simulink model "Journal2022"  (R2018a)
settings: Solver=VariableStepAuto  StartTime=0.0  StopTime=20  FixedStep=1e-6  MinStep=1e-3  RelTol=1e-3  EnableMultiTasking=on
PreLoadFcn:
  | if count(py.sys.path,'') == 0
  | insert(py.sys.path,int32(0),'');
  | end
InitFcn:
  | clear all
  | close all
  | Variables_Journal2022
StopFcn:
  | %Figures_Test_Pytorch_simulink
values from neighbouring files (symbols this model uses):
  den_Tdel = [0 0.2]    [TestKalm.mat]    (also in Variables_Journal2022.m)
  Fz_routa = 7840    [TestKalm.mat]    (also in Variables_Journal2022.m)
  G1 = -4.99    [Variables_Journal2022.m]
  G2 = -18.43    [Variables_Journal2022.m]
  G3 = -65.62    [Variables_Journal2022.m]
  lambda_dummy = [0 0.000200040008002 0.000400080016003 0.000600120024005 0.000800160032006 0.00100020004001 0.00120024004801 0.00140028005601 0.00160032006401 0.00180036007201 0.00200040008002 0.00220044008802 ... (5000 elements, 1x5000)]    [TestKalm.mat]    (also in Variables_Journal2022.m = linspace(0, 1, num_samples_lambda))
  Massa_drone_eq = 800    [TestKalm.mat]    (also in Variables_Journal2022.m)
  ML_sample_time = 0.005    [TestKalm.mat]    (also in Variables_Journal2022.m)
  Momento_inerzia = 0.45    [TestKalm.mat]    (also in Variables_Journal2022.m)
  omega0 = 266.666666667    [TestKalm.mat]    (also in Variables_Journal2022.m)
  PI_ki = 20    [TestKalm.mat]    (also in Variables_Journal2022.m)
  PI_kp = 0.5    [TestKalm.mat]    (also in Variables_Journal2022.m)
  Raggio_pneumatico = 0.3    [TestKalm.mat]    (also in Variables_Journal2022.m)
  Sample_time = 0.005    [TestKalm.mat]    (also in Variables_Journal2022.m)
  v0 = 80    [TestKalm.mat]    (also in Variables_Journal2022.m)
  v_min_stop = 15    [Variables_Journal2022.m]
  v_state_space_A = [-200  -10000; 1  0]    [TestKalm.mat]    (also in Variables_Journal2022.m = Av)
  v_state_space_B = [1 0]    [TestKalm.mat]    (also in Variables_Journal2022.m = Bv)
  v_state_space_C = [10000  0; 1  0; 0  1]    [TestKalm.mat]    (also in Variables_Journal2022.m = [Cv; eye(2)])
  v_state_space_D = [0 0 0]    [TestKalm.mat]    (also in Variables_Journal2022.m = [Dv; 0;0])
  v_state_space_init = [0 0.008]    [TestKalm.mat]    (also in Variables_Journal2022.m = [inv(Av)*-Bv*v0])
  w_state_Space_A = [-200  -10000; 1  0]    [TestKalm.mat]    (also in Variables_Journal2022.m = Aw)
  w_state_Space_B = [1 0]    [TestKalm.mat]    (also in Variables_Journal2022.m = Bw)
  w_state_Space_C = [10000  0; 1  0; 0  1]    [TestKalm.mat]    (also in Variables_Journal2022.m = [Cw; eye(2)])
  w_state_Space_D = [0 0 0]    [TestKalm.mat]    (also in Variables_Journal2022.m = [Dw; 0;0])
  w_state_space_init = [0 0.0266666666667]    [TestKalm.mat]    (also in Variables_Journal2022.m = [inv(Aw)*-Bw*omega0])
undefined symbols (not defined in the file or in its folder): sigbuilder_block
libraries: simulink x5, ctrlSharedLib x1
settings Model: Creator=Francesco  LastModifiedBy=Francesco Crocetti
settings DataIOCC: LimitDataPoints=on  SaveFormat=Array
settings OptimizationCC: LifeSpan=inf
settings DebuggingCC: SolverPrmCheckMsg=warning  SFUnexpectedBacktrackingDiag=warning  SFNoUnconditionalDefaultTransitionDiag=warning  SFExecutionAtInitializationDiag=none
settings HardwareCC: ProdBitPerPointer=32  ProdBitPerSizeT=32  ProdBitPerPtrDiffT=32  ProdLargestAtomicFloat=None  ProdIntDivRoundTo=Undefined  ProdEndianess=Unspecified  ProdWordSize=32  ProdHWDeviceType=32-bit Generic
settings ModelReferenceCC: PropagateSignalLabelsOutOfModel=off
settings CodeAppCC: StateflowObjectComments=on
settings GRTTargetCC: TargetLangStandard=C89/C90 (ANSI)  GeneratePreprocessorConditionals=Disable all
settings ConfigComp: CovMetricSettings=dw  CovHtmlReporting=on  CovSaveCumulativeToWorkspaceVar=on  CovSaveSingleToWorkspaceVar=on  CovExternalEMLEnable=off  CovSFcnEnable=off

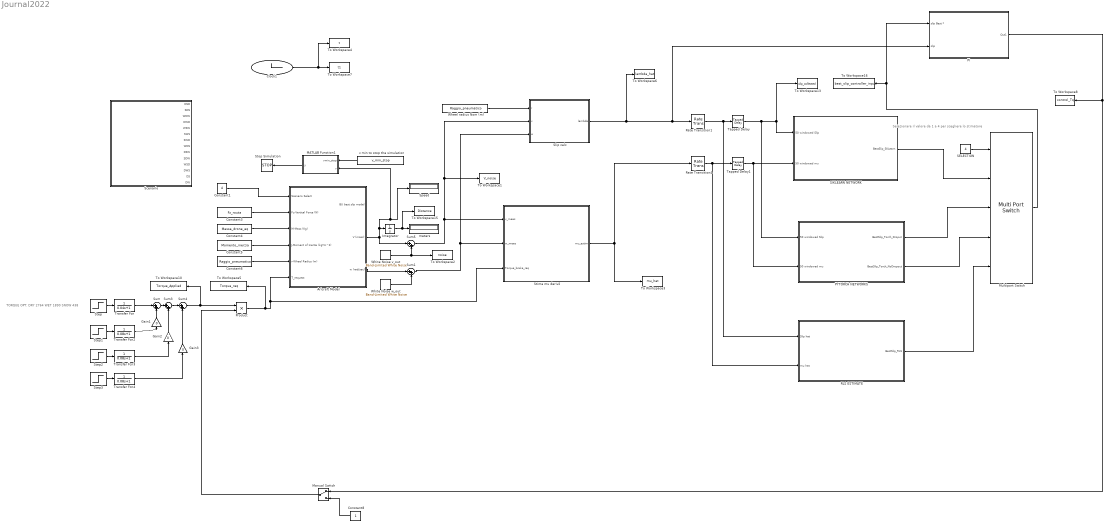
== system Journal2022 ==
  note: TORQUE OPT: DRY 2764 WET 1890 SNOW 438
  note: Selezionare il valore da 1 a 4 per scegliere lo stimatore
  Aricraft Model : Subsystem
  Clock1 : Clock
  Constant1 : Constant  Value=4
  Constant3 : Constant  Value=Fz_routa
  Constant4 : Constant  Value=Massa_drone_eq
  Constant5 : Constant  Value=Momento_inerzia
  Constant6 : Constant  Value=Raggio_pneumatico
  Constant8 : Constant
  Gain1 : Gain  Gain=0
  Gain2 : Gain  Gain=0
  Gain3 : Gain  Gain=0
  Integrator : Integrator
  MATLAB Function1 : MATLAB Function  TreatAsAtomicUnit=on
  Manual Switch : ManualSwitch
  Multiport Switch : MultiPortSwitch  DataPortOrder=Specify indices  Inputs=4  DataPortIndices={1,2,3,4}  DiagnosticForDefault=None  OutDataTypeStr=double  RndMeth=Round
  "PI " : Subsystem
  PYTORCH NETWORKS : Subsystem
  Product : Product
  RLS ESTIMATE : Subsystem
  Rate Transition1 : RateTransition  OutPortSampleTime=ML_sample_time
  Rate Transition4 : RateTransition  OutPortSampleTime=ML_sample_time
  SELECTION : Constant  Value=4
  SIKLEARN NETWORK : Subsystem
  "Scenario " : Subsystem  Tag=STV Subsys  LoadFcn=sigbuilder_block('load');  StartFcn=sigbuilder_block('start');  StopFcn=sigbuilder_block('stop');  ClipboardFcn=sigbuilder_block('clipboard');  mask(Sigbuilder block){tuvar=[0:10]}
      mask help: Simulink:masks:SigbuilderBlock_MD
      mask init:
      | if ~strcmp(get_param(bdroot(gcbh),'SimulationStatus'),'stopped') tuvar = sigbuilder_block('maskInit'); end
      settings: CopyFcn=sigbuilder_block('copy');  DeleteFcn=sigbuilder_block('delete');  ModelCloseFcn=sigbuilder_block('modelClose');  PreSaveFcn=sigbuilder_block('preSave');  PauseFcn=sigbuilder_block('pause');  ContinueFcn=sigbuilder_block('continue');  NameChangeFcn=sigbuilder_block('namechange');  OpenFcn=sigbuilder_block('open',[48.75 0 1391.25 690 ]);  CloseFcn=sigbuilder_block('close');
      mask Display: plot(0, 0, 100, 100,[2, 2, 32, 32, 2], [68, 8, 8, 68, 68],[32, 2], [38, 38], [32, 19, 2],[53, 60, 44], [32, 17, 17, 2],[16, 16, 31, 31]);txt = getActiveGroup(gcbh);text(2, 100, txt,'verticalAlignment', 'top');
  Slip calc : MATLAB Function  TreatAsAtomicUnit=on
  Speed : Display
  Step : Step  Time=0  After=3764  SampleTime=0
  Step1 : Step  Time=2  After=-500  SampleTime=0
  Step2 : Step  Time=4  After=-500  SampleTime=0
  Step3 : Step  Time=6  After=-500  SampleTime=0
  Stima mu deriv2 : Subsystem
  Stop Simulation : Stop
  Sum{,1,3..5} (5 alike) : Sum  Inputs=|++
  Tapped Delay : simulink/Discrete/Tapped Delay  vinit=0.2  samptime=-1  NumDelays=50  DelayOrder=Newest  includeCurrent=off
  Tapped Delay1 : simulink/Discrete/Tapped Delay  vinit=1  samptime=-1  NumDelays=50  DelayOrder=Newest  includeCurrent=off
  To Workspace1 : ToWorkspace  VariableName=V_noise  SampleTime=-1
  To Workspace10 : ToWorkspace  VariableName=Torque_Applied  SampleTime=-1
  To Workspace13 : ToWorkspace  VariableName=slip_collected  SampleTime=-1
  To Workspace15 : ToWorkspace  VariableName=Distance  SampleTime=-1
  To Workspace16 : ToWorkspace  VariableName=best_slip_controller_input  SampleTime=-1
  To Workspace2 : ToWorkspace  VariableName=noise  SampleTime=-1
  To Workspace3 : ToWorkspace  VariableName=mu_hat  SampleTime=-1
  To Workspace4 : ToWorkspace  VariableName=t  SampleTime=-1
  To Workspace5 : ToWorkspace  VariableName=Torque_req  SampleTime=-1
  To Workspace6 : ToWorkspace  VariableName=lambda_hat  SampleTime=-1
  To Workspace7 : ToWorkspace  VariableName=t1  SampleTime=Sample_time
  To Workspace8 : ToWorkspace  VariableName=control_Tq  SampleTime=-1
  Transfer Fcn : TransferFcn  Denominator=[0.04 1]
  Transfer Fcn2 : TransferFcn  Denominator=[0.08 1]
  Transfer Fcn3 : TransferFcn  Denominator=[0.08 1]
  Transfer Fcn4 : TransferFcn  Denominator=[0.08 1]
  Wheel radius Nom (m) : Constant  Value=Raggio_pneumatico
  White Noise v_out : simulink/Sources/Band-Limited White Noise  Cov=Pow_WN_vout_model  Ts=Sample_time  seed=[75893]
  White Noise w_out : simulink/Sources/Band-Limited White Noise  Cov=Pow_WN_wout_model  Ts=Sample_time  seed=[17523]
  meters : Display
  v min to stop the simulation : Constant  Value=v_min_stop
  wires:
  Integrator/1 -> To Workspace15/1, meters/1
  Constant6/1 -> Aricraft Model/5(r-Wheel Radius (m))
  Wheel radius Nom (m)/1 -> Slip calc/1(r)
  Constant4/1 -> Aricraft Model/3(" M-Mass (Kg)")
  Constant5/1 -> Aricraft Model/4(J-Moment of Inertia (‎kg*m^2))
  Sum5/1 -> Stima mu deriv2/1(v_meas), To Workspace1/1, Slip calc/2(v)
  Rate Transition4/1 -> RLS ESTIMATE/2(mu hat), Tapped Delay1/1
  Aricraft Model/3(w (rad/sec)) -> Sum1/1
  Sum1/1 -> Stima mu deriv2/2(w_meas), Slip calc/3(w)
  Clock1/1 -> To Workspace7/1, To Workspace4/1
  Transfer Fcn/1 -> Sum/1
  Step/1 -> Transfer Fcn/1
  Sum3/1 -> Sum4/1
  Transfer Fcn2/1 -> Gain1/1
  Step1/1 -> Transfer Fcn2/1
  Step2/1 -> Transfer Fcn3/1
  Transfer Fcn4/1 -> Gain3/1
  Transfer Fcn3/1 -> Gain2/1
  Sum/1 -> Sum3/1
  Step3/1 -> Transfer Fcn4/1
  Stima mu deriv2/1("mu_estim ") -> To Workspace3/1, Rate Transition4/1
  Slip calc/1(lambda) -> To Workspace6/1, "PI "/2("slip "), Rate Transition1/1
  Sum4/1 -> To Workspace10/1, Product/1
  Gain1/1 -> Sum/2
  Gain2/1 -> Sum3/2
  Gain3/1 -> Sum4/2
  Constant3/1 -> Aricraft Model/2(Fz-Vertical Force (N))
  Tapped Delay/1 -> PYTORCH NETWORKS/1(50 windowed Slip), SIKLEARN NETWORK/1(50 windowed Slip), To Workspace13/1
  White Noise v_out/1 -> Sum5/2, To Workspace2/1
  White Noise w_out/1 -> Sum1/2
  Tapped Delay1/1 -> SIKLEARN NETWORK/2(50 windowed mu), PYTORCH NETWORKS/2(50 windowed mu)
  Product/1 -> To Workspace5/1, Stima mu deriv2/3(Torque_brake_req), Aricraft Model/6(T_request)
  Rate Transition1/1 -> RLS ESTIMATE/1(" Slip hat"), Tapped Delay/1
  Constant8/1 -> Manual Switch/2
  Manual Switch/1 -> Product/2
  "PI "/1(Out1) -> Manual Switch/1, To Workspace8/1
  Multiport Switch/1 -> To Workspace16/1, "PI "/1("slip Best * ")
  PYTORCH NETWORKS/1(BestSlip_Torch_Droput) -> Multiport Switch/3
  PYTORCH NETWORKS/2(BestSlip_Torch_NoDropout) -> Multiport Switch/4
  MATLAB Function1/1(y) -> Stop Simulation/1
  Aricraft Model/2(V (msec)) -> Sum5/1, MATLAB Function1/2(v), Speed/1, Integrator/1
  v min to stop the simulation/1 -> MATLAB Function1/1(vmin_stop)
  RLS ESTIMATE/1("BestSlip_RLS ") -> Multiport Switch/5
  SELECTION/1 -> Multiport Switch/1
  SIKLEARN NETWORK/1(BestSlip_SKLearn) -> Multiport Switch/2
  Constant1/1 -> Aricraft Model/1("Scenario Select ")

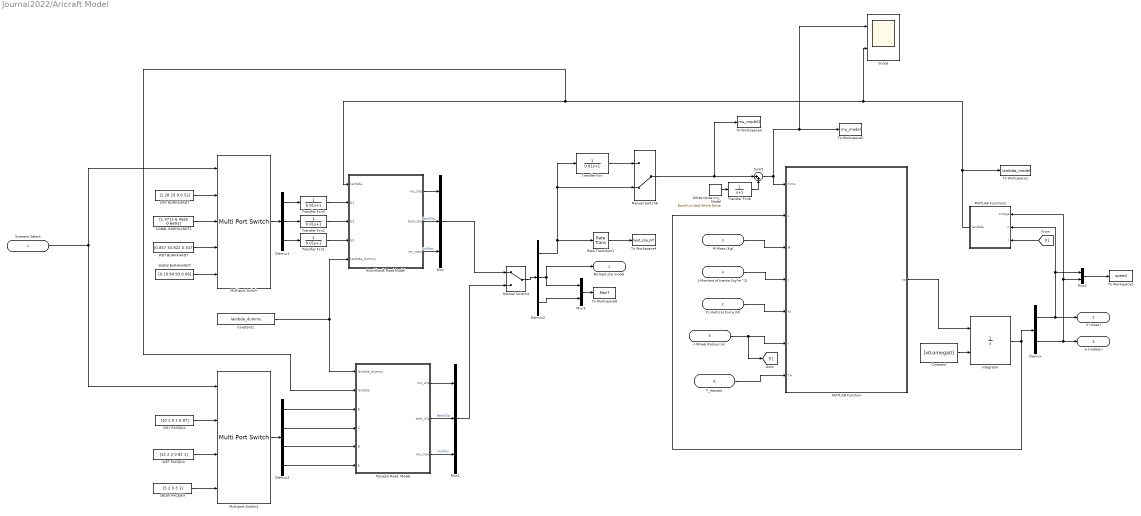
== system Journal2022/Aricraft Model ==
  "Scenario Select " : Inport
  Fz-Vertical Force (N) : Inport  Port=2
  " M-Mass (Kg)" : Inport  Port=3
  J-Moment of Inertia (‎kg*m^2) : Inport  Port=4
  r-Wheel Radius (m) : Inport  Port=5
  T_request : Inport  Port=6
  Burchkardt Road Model : MATLAB Function  TreatAsAtomicUnit=on
  COBBL BURHKARDT1 : Constant  Value=[1.3713 6.4565 0.6691]
  Constant : Constant  Value=[v0,omega0]
  Constant1 : Constant  Value=lambda_dummy
  DRY BURHKARDT : Constant  Value=[1.28 23.9 0.52]
  DRY PACEJKA : Constant  Value=[10 1.9 1 0.97]
  Demux : Demux  Outputs=2
  Demux1 : Demux  Outputs=3
  Demux2 : Demux
  Demux3 : Demux  Outputs=3
  Integrator : Integrator  InitialConditionSource=external  InitialCondition=[v0,omega0]  LimitOutput=on  LowerSaturationLimit=0
  MATLAB Function : MATLAB Function  TreatAsAtomicUnit=on
  MATLAB Function2 : MATLAB Function  TreatAsAtomicUnit=on
  Manual Switch4 : ManualSwitch
  Manual Switch6 : ManualSwitch  CurrentSetting=0
  Multiport Switch : MultiPortSwitch  DataPortOrder=Specify indices  Inputs=4  DataPortIndices={1,2,3,4}  DiagnosticForDefault=None
  Multiport Switch1 : MultiPortSwitch  DataPortOrder=Specify indices  Inputs=4  DiagnosticForDefault=None
  Mux : Mux  Inputs=3
  Mux1 : Mux  Inputs=3
  Mux2 : Mux  Inputs=2
  Mux3 : Mux  Inputs=2
  Pacejka Road  Model : MATLAB Function  TreatAsAtomicUnit=on
  Rate Transition1 : RateTransition  OutPortSampleTime=ML_sample_time
  SNOW BURHKARDT : Constant  Value=[0.19 94.93 0.06]
  SNOW PACEJKA : Constant  Value=[5 2 0.3 1]
  Scope : Scope  NumInputPorts=2
  Sum5 : Sum  Inputs=|++
  To Workspace1 : ToWorkspace  VariableName=lambda_model  SampleTime=-1
  To Workspace2 : ToWorkspace  VariableName=speed  SampleTime=-1
  To Workspace3 : ToWorkspace  VariableName=mu_model1  SampleTime=-1
  To Workspace4 : ToWorkspace  VariableName=best_slip_GT  SampleTime=-1
  To Workspace5 : ToWorkspace  VariableName=mu_model  SampleTime=-1
  To Workspace8 : ToWorkspace  VariableName=MaxT  SampleTime=-1
  Transfer Fcn{,1..3} (4 alike) : TransferFcn  Denominator=[0.01 1]
  Transfer Fcn6 : TransferFcn  Denominator=[1 1]
  WET BURHKARDT : Constant  Value=[0.857 33.822 0.347]
  WET PACEJKA : Constant  Value=[12 2.3 0.82 1]
  "White Noise mu_Model " : simulink/Sources/Band-Limited White Noise  Cov=Pow_WN_model  Ts=Sample_time  seed=[15523]
  BU best slip model : Outport
  V (msec) : Outport  Port=2
  w (rad/sec) : Outport  Port=3
  wires:
  MATLAB Function/1(xp) -> Integrator/1
  T_request/1 -> MATLAB Function/7(Tw)
  Constant/1 -> Integrator/2
  Integrator/1 -> Demux/1, MATLAB Function/2(x)
  " M-Mass (Kg)"/1 -> MATLAB Function/3(M)
  J-Moment of Inertia (‎kg*m^2)/1 -> MATLAB Function/4(J)
  Fz-Vertical Force (N)/1 -> MATLAB Function/5(Fz)
  r-Wheel Radius (m)/1 -> [r], MATLAB Function/6(r)
  Demux/1 -> V (msec)/1, MATLAB Function2/2(v), Mux2/1
  Demux/2 -> w (rad/sec)/1, Mux2/2, MATLAB Function2/1(omega)
  Mux2/1 -> To Workspace2/1
  Multiport Switch/1 -> Demux1/1
  Demux2/3 -> Pacejka Road  Model/5(D)
  Demux2/2 -> Pacejka Road  Model/4(C)
  Demux2/1 -> Pacejka Road  Model/3(B)
  Demux2/4 -> Pacejka Road  Model/6(E)
  DRY PACEJKA/1 -> Multiport Switch1/2
  Multiport Switch1/1 -> Demux2/1
  WET PACEJKA/1 -> Multiport Switch1/3
  SNOW PACEJKA/1 -> Multiport Switch1/4
  "White Noise mu_Model "/1 -> Transfer Fcn6/1
  MATLAB Function2/1(lambda) -> To Workspace1/1, Scope/2, Pacejka Road  Model/2(lambda), Burchkardt Road Model/1(lambda)
  Constant1/1 -> Pacejka Road  Model/1(lambda_dummy), Burchkardt Road Model/5(lambda_dummy)
  Sum5/1 -> Scope/1, To Workspace5/1, MATLAB Function/1(mmu)
  Manual Switch6/1 -> To Workspace3/1, Sum5/1
  DRY BURHKARDT/1 -> Multiport Switch/2
  WET BURHKARDT/1 -> Multiport Switch/4
  Transfer Fcn6/1 -> Sum5/2
  Burchkardt Road Model/1(mu_slip) -> Mux/1
  Burchkardt Road Model/2(best_slip) -> Mux/2  "BestSlip"
  Burchkardt Road Model/3(mu_max) -> Mux/3  "muMax"
  Pacejka Road  Model/3(mu_max) -> Mux1/3  "muMax"
  Pacejka Road  Model/1(mu_slip) -> Mux1/1
  Pacejka Road  Model/2(best_slip) -> Mux1/2  "BestSlip"
  Mux/1 -> Manual Switch4/1
  Mux1/1 -> Manual Switch4/2
  Manual Switch4/1 -> Demux3/1
  Demux3/3 -> Mux3/2
  Mux3/1 -> To Workspace8/1
  Demux3/2 -> BU best slip model/1, Mux3/1
  Transfer Fcn/1 -> Manual Switch6/1
  Demux3/1 -> Rate Transition1/1, Transfer Fcn/1, Manual Switch6/2
  COBBL BURHKARDT1/1 -> Multiport Switch/3
  SNOW BURHKARDT/1 -> Multiport Switch/5
  "Scenario Select "/1 -> Multiport Switch1/1, Multiport Switch/1
  Demux1/1 -> Transfer Fcn3/1
  Demux1/3 -> Transfer Fcn1/1
  Demux1/2 -> Transfer Fcn2/1
  Transfer Fcn1/1 -> Burchkardt Road Model/4(b3)
  Transfer Fcn2/1 -> Burchkardt Road Model/3(b2)
  Transfer Fcn3/1 -> Burchkardt Road Model/2(b1)
  [r] -> MATLAB Function2/3(r)
  Rate Transition1/1 -> To Workspace4/1

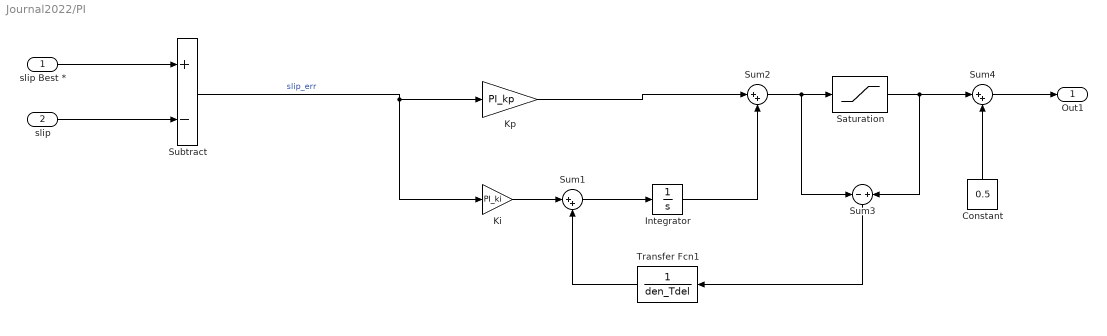
== system Journal2022/PI  ==
  "slip Best * " : Inport
  "slip " : Inport  Port=2
  Constant : Constant  Value=0.5
  Integrator : Integrator
  Ki : Gain  Gain=PI_ki
  "Kp " : Gain  Gain=PI_kp
  Saturation : Saturate
  Subtract : Sum  Inputs=+-
  Sum1 : Sum  Inputs=|++
  Sum2 : Sum  Inputs=|++
  Sum3 : Sum  Inputs=-|+
  Sum4 : Sum  Inputs=|++
  Transfer Fcn1 : TransferFcn  Denominator=den_Tdel
  Out1 : Outport
  wires:
  Sum3/1 -> Transfer Fcn1/1
  Integrator/1 -> Sum2/2
  Sum1/1 -> Integrator/1
  Sum2/1 -> Sum3/1, Saturation/1
  Ki/1 -> Sum1/1
  Transfer Fcn1/1 -> Sum1/2
  Subtract/1 -> Ki/1, "Kp "/1  "slip_err"
  "Kp "/1 -> Sum2/1
  Saturation/1 -> Sum4/1, Sum3/2
  "slip Best * "/1 -> Subtract/1
  "slip "/1 -> Subtract/2
  Sum4/1 -> Out1/1
  Constant/1 -> Sum4/2

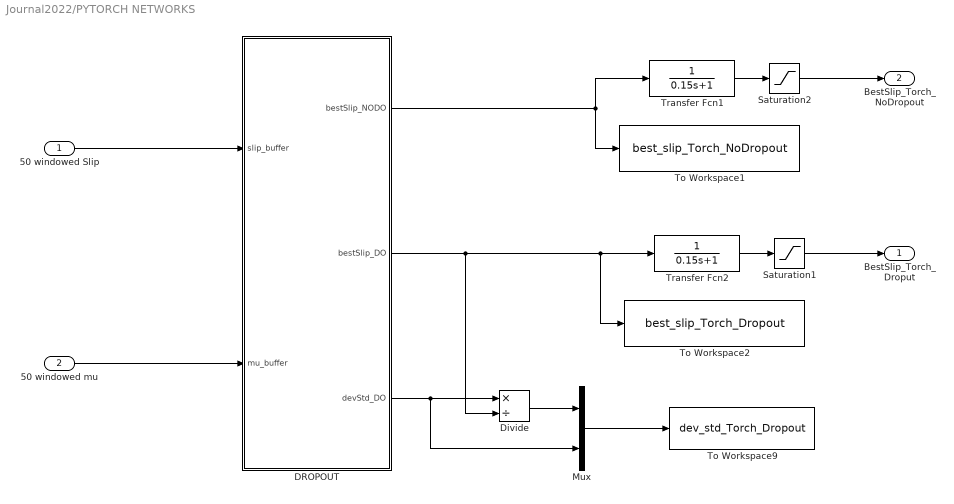
== system Journal2022/PYTORCH NETWORKS ==
  50 windowed Slip : Inport
  50 windowed mu : Inport  Port=2
  " DROPOUT" : MATLAB Function  TreatAsAtomicUnit=on
  Divide : Product  Inputs=*/
  Mux : Mux  Inputs=2
  Saturation1 : Saturate  UpperLimit=1  LowerLimit=0.001
  Saturation2 : Saturate  UpperLimit=1  LowerLimit=0.001
  To Workspace1 : ToWorkspace  VariableName=best_slip_Torch_NoDropout  SampleTime=-1
  To Workspace2 : ToWorkspace  VariableName=best_slip_Torch_Dropout  SampleTime=-1
  To Workspace9 : ToWorkspace  VariableName=dev_std_Torch_Dropout  SampleTime=-1
  Transfer Fcn1 : TransferFcn  Denominator=[0.15 1]
  Transfer Fcn2 : TransferFcn  Denominator=[0.15 1]
  BestSlip_Torch_Droput : Outport
  BestSlip_Torch_NoDropout : Outport  Port=2
  wires:
  " DROPOUT"/1(bestSlip_NODO) -> To Workspace1/1, Transfer Fcn1/1
  " DROPOUT"/3(devStd_DO) -> Mux/2, Divide/1
  Transfer Fcn1/1 -> Saturation2/1
  50 windowed Slip/1 -> " DROPOUT"/1(slip_buffer)
  50 windowed mu/1 -> " DROPOUT"/2(mu_buffer)
  Divide/1 -> Mux/1
  Mux/1 -> To Workspace9/1
  Saturation2/1 -> BestSlip_Torch_NoDropout/1
  Transfer Fcn2/1 -> Saturation1/1
  " DROPOUT"/2(bestSlip_DO) -> Divide/2, To Workspace2/1, Transfer Fcn2/1
  Saturation1/1 -> BestSlip_Torch_Droput/1

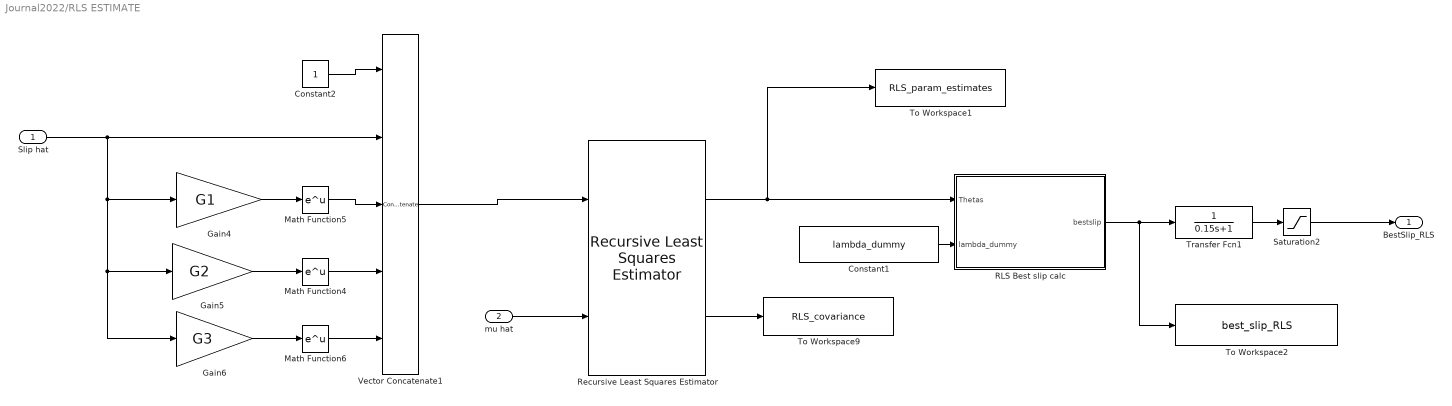
== system Journal2022/RLS ESTIMATE ==
  " Slip hat" : Inport
  mu hat : Inport  Port=2
  Constant1 : Constant  Value=lambda_dummy
  Constant2 : Constant
  Gain4 : Gain  Gain=G1
  Gain5 : Gain  Gain=G2
  Gain6 : Gain  Gain=G3
  Math Function4 : Math  SaturateOnIntegerOverflow=on
  Math Function5 : Math  SaturateOnIntegerOverflow=on
  Math Function6 : Math  SaturateOnIntegerOverflow=on
  RLS Best slip calc : MATLAB Function  TreatAsAtomicUnit=on
  Recursive Least Squares Estimator : ctrlSharedLib/Recursive Least Squares Estimator  InitialEstimateSource=Internal  InitialParameterData=RLS_Init_param_values  P0=RLS_Ro_Covar_Mat  EstimationMethod=Forgetting Factor  AdaptationParameter=RLS_Forgetting_factor  HasTimeVaryingAdaptationParameter=off  NormalizationBias=eps  OutputError=off  OutputP=on  AddEnablePort=off  Ts=ML_sample_time
      settings: SourceProductName=Control System Toolbox  SourceProductBaseCode=CT
  Saturation2 : Saturate  UpperLimit=1  LowerLimit=0.001
  To Workspace1 : ToWorkspace  VariableName=RLS_param_estimates  SampleTime=-1
  To Workspace2 : ToWorkspace  VariableName=best_slip_RLS  SampleTime=-1
  To Workspace9 : ToWorkspace  VariableName=RLS_covariance  SampleTime=-1
  Transfer Fcn1 : TransferFcn  Denominator=[0.15 1]
  Vector Concatenate1 : Concatenate  NumInputs=5
  "BestSlip_RLS " : Outport
  wires:
  Constant1/1 -> RLS Best slip calc/2(lambda_dummy)
  Recursive Least Squares Estimator/1 -> To Workspace1/1, RLS Best slip calc/1(Thetas)
  Vector Concatenate1/1 -> Recursive Least Squares Estimator/1
  Math Function6/1 -> Vector Concatenate1/5
  Gain4/1 -> Math Function5/1
  " Slip hat"/1 -> Gain6/1, Gain5/1, Gain4/1, Vector Concatenate1/2
  Math Function5/1 -> Vector Concatenate1/3
  Gain6/1 -> Math Function6/1
  Gain5/1 -> Math Function4/1
  Math Function4/1 -> Vector Concatenate1/4
  Constant2/1 -> Vector Concatenate1/1
  mu hat/1 -> Recursive Least Squares Estimator/2
  Recursive Least Squares Estimator/2 -> To Workspace9/1
  Transfer Fcn1/1 -> Saturation2/1
  RLS Best slip calc/1(bestslip) -> To Workspace2/1, Transfer Fcn1/1
  Saturation2/1 -> "BestSlip_RLS "/1

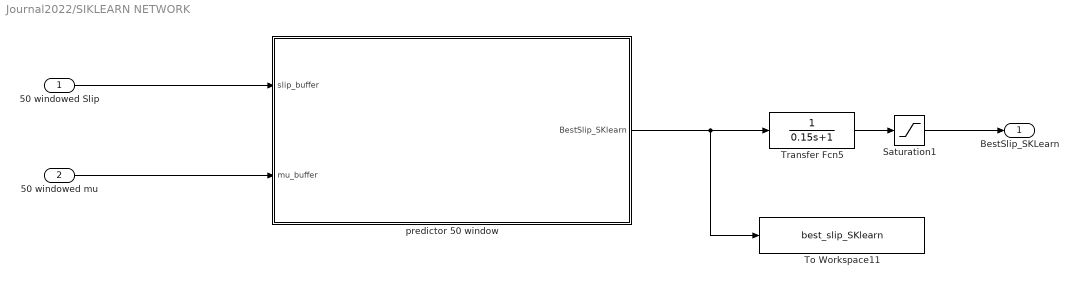
== system Journal2022/SIKLEARN NETWORK ==
  50 windowed Slip : Inport
  50 windowed mu : Inport  Port=2
  Saturation1 : Saturate  UpperLimit=1  LowerLimit=0.001
  To Workspace11 : ToWorkspace  VariableName=best_slip_SKlearn  SampleTime=-1
  Transfer Fcn5 : TransferFcn  Denominator=[0.15 1]
  predictor 50 window : MATLAB Function  TreatAsAtomicUnit=on
  BestSlip_SKLearn : Outport
  wires:
  50 windowed Slip/1 -> predictor 50 window/1(slip_buffer)
  50 windowed mu/1 -> predictor 50 window/2(mu_buffer)
  predictor 50 window/1(BestSlip_SKlearn) -> To Workspace11/1, Transfer Fcn5/1
  Transfer Fcn5/1 -> Saturation1/1
  Saturation1/1 -> BestSlip_SKLearn/1

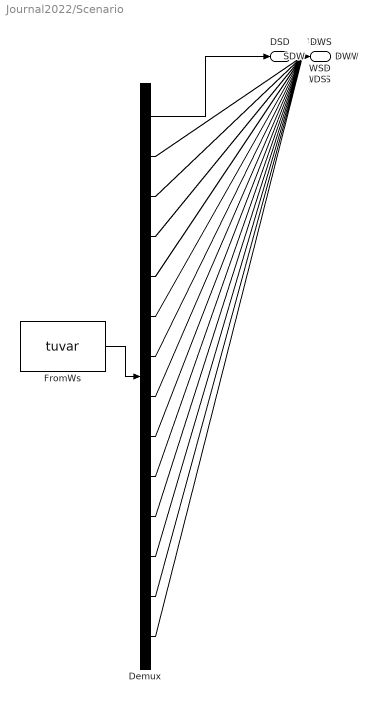
== system Journal2022/Scenario  ==
  Demux : Demux  Tag=STV Demux  Outputs=14
  FromWs : FromWorkspace  Tag=STV FromWs  VariableName=tuvar  SampleTime=0
      SigBuilderData=|
      | common.afterFinalStr = 'Extrapolate'
      | common.sampleTime = 0
      | dataSet.timeRange = [0 20]
      | dataSet.name = 'Group 1'
      | sbobj.Groups.Name = 'Group 1'
      | sbobj.Groups.Signals(1).Name = 'DSD'
      | sbobj.Groups.Signals(1).XData = [0 2 2 4 4 20]
      | sbobj.Groups.Signals(1).YData = [1 1 4 4 1 1]
      | sbobj.Groups.Signals(2).Name = 'SDS'
      | sbobj.Groups.Signals(2).XData = [0 2 2 6 6 20]
      | sbobj.Groups.Signals(2).YData = [4 4 1 1 4 4]
      | sbobj.Groups.Signals(3).Name = 'WDW'
      | sbobj.Groups.Signals(3).XData = [0 3 3 6 6 20]
      | sbobj.Groups.Signals(3).YData = [3 3 1 1 3 3]
      | sbobj.Groups.Signals(4).Name = 'DWD'
      | sbobj.Groups.Signals(4).XData = [0 3 3 6 6 20]
      | sbobj.Groups.Signals(4).YData = [1 1 3 3 1 1]
      | sbobj.Groups.Signals(5).Name = 'WSW'
      | sbobj.Groups.Signals(5).XData = [0 4 4 7 7 20]
      | sbobj.Groups.Signals(5).YData = [3 3 4 4 3 3]
      | sbobj.Groups.Signals(6).Name = 'SWS'
      | sbobj.Groups.Signals(6).XData = [0 4 4 8 8 20]
      | sbobj.Groups.Signals(6).YData = [4 4 3 3 4 4]
      | sbobj.Groups.Signals(7).Name = 'SWD'
      | sbobj.Groups.Signals(7).XData = [0 3 3 6 6 20]
      | sbobj.Groups.Signals(7).YData = [4 4 3 3 1 1]
      | sbobj.Groups.Signals(8).Name = 'WDS'
      | sbobj.Groups.Signals(8).XData = [0 3 3 5 5 20]
      | sbobj.Groups.Signals(8).YData = [3 3 1 1 4 4]
      | sbobj.Groups.Signals(9).Name = 'DSW'
      | sbobj.Groups.Signals(9).XData = [0 3 3 6 6 20]
      | sbobj.Groups.Signals(9).YData = [1 1 4 4 3 3]
      | sbobj.Groups.Signals(10).Name = 'SDW'
      | sbobj.Groups.Signals(10).XData = [0 4 4 7 7 20]
      | sbobj.Groups.Signals(10).YData = [4 4 1 1 3 3]
      | sbobj.Groups.Signals(11).Name = 'WSD'
      | sbobj.Groups.Signals(11).XData = [0 4 4 7 7 20]
      | sbobj.Groups.Signals(11).YData = [3 3 4 4 1 1]
      | sbobj.Groups.Signals(12).Name = 'DWS'
      | sbobj.Groups.Signals(12).XData = [0 3 3 5 5 20]
      | sbobj.Groups.Signals(12).YData = [1 1 3 3 4 4]
      | sbobj.Groups.Signals(13).Name = 'DS'
      | sbobj.Groups.Signals(13).XData = [0 3 3 20]
      | sbobj.Groups.Signals(13).YData = [1 1 4 4]
      | sbobj.Groups.Signals(14).Name = 'DW'
      | sbobj.Groups.Signals(14).XData = [0 3 3 20]
      | sbobj.Groups.Signals(14).YData = [1 1 3 3]
      | sbobj.Groups.TimeRange = [0 20]
  DSD : Outport  Tag=STV Outport
  SDS : Outport  Tag=STV Outport  Port=2
  WDW : Outport  Tag=STV Outport  Port=3
  DWD : Outport  Tag=STV Outport  Port=4
  WSW : Outport  Tag=STV Outport  Port=5
  SWS : Outport  Tag=STV Outport  Port=6
  SWD : Outport  Tag=STV Outport  Port=7
  WDS : Outport  Tag=STV Outport  Port=8
  DSW : Outport  Tag=STV Outport  Port=9
  SDW : Outport  Tag=STV Outport  Port=10
  WSD : Outport  Tag=STV Outport  Port=11
  DWS : Outport  Tag=STV Outport  Port=12
  DS : Outport  Tag=STV Outport  Port=13
  DW : Outport  Tag=STV Outport  Port=14
  wires:
  Demux/1 -> DSD/1
  FromWs/1 -> Demux/1
  Demux/2 -> SDS/1
  Demux/3 -> WDW/1
  Demux/4 -> DWD/1
  Demux/5 -> WSW/1
  Demux/6 -> SWS/1
  Demux/7 -> SWD/1
  Demux/8 -> WDS/1
  Demux/9 -> DSW/1
  Demux/10 -> SDW/1
  Demux/11 -> WSD/1
  Demux/12 -> DWS/1
  Demux/13 -> DS/1
  Demux/14 -> DW/1

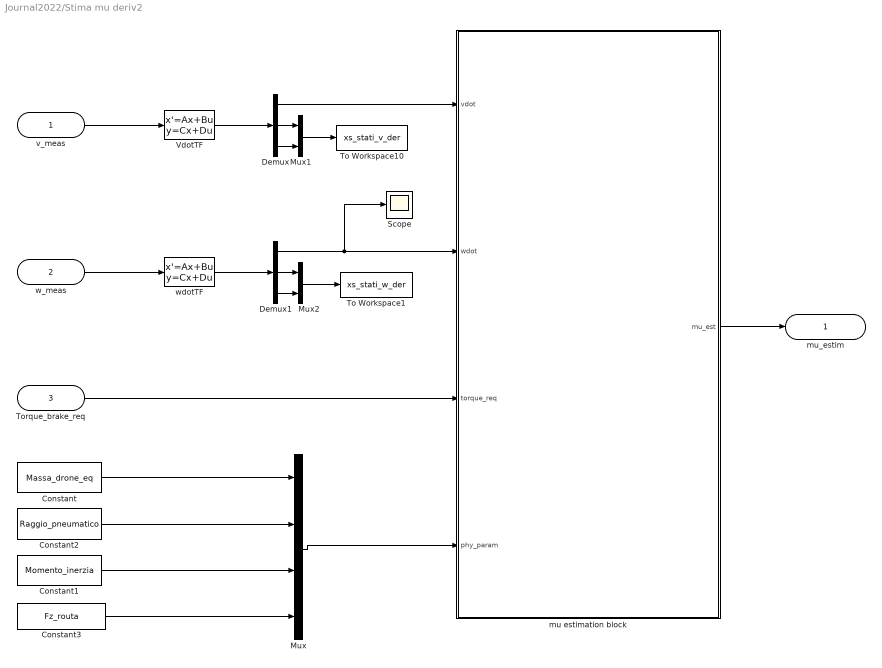
== system Journal2022/Stima mu deriv2 ==
  v_meas : Inport
  w_meas : Inport  Port=2
  Torque_brake_req : Inport  Port=3
  Constant : Constant  Value=Massa_drone_eq
  Constant1 : Constant  Value=Momento_inerzia
  Constant2 : Constant  Value=Raggio_pneumatico
  Constant3 : Constant  Value=Fz_routa
  Demux : Demux  Outputs=3
  Demux1 : Demux  Outputs=3
  Mux : Mux
  Mux1 : Mux  Inputs=2
  Mux2 : Mux  Inputs=2
  Scope : Scope
  To Workspace1 : ToWorkspace  VariableName=xs_stati_w_der  SampleTime=Sample_time
  To Workspace10 : ToWorkspace  VariableName=xs_stati_v_der  SampleTime=Sample_time
  "VdotTF " : StateSpace  A=v_state_space_A  B=v_state_space_B  C=v_state_space_C  D=v_state_space_D  InitialCondition=v_state_space_init
  mu estimation block : MATLAB Function  TreatAsAtomicUnit=on
  "wdotTF " : StateSpace  A=w_state_Space_A  B=w_state_Space_B  C=w_state_Space_C  D=w_state_Space_D  InitialCondition=w_state_space_init
  "mu_estim " : Outport
  wires:
  mu estimation block/1(mu_est) -> "mu_estim "/1
  Torque_brake_req/1 -> mu estimation block/3(torque_req)
  Mux/1 -> mu estimation block/4(phy_param)
  Constant/1 -> Mux/1
  "VdotTF "/1 -> Demux/1
  Demux/1 -> mu estimation block/1(vdot)
  v_meas/1 -> "VdotTF "/1
  Demux/2 -> Mux1/1
  Demux/3 -> Mux1/2
  Mux1/1 -> To Workspace10/1
  Demux1/1 -> Scope/1, mu estimation block/2(wdot)
  Demux1/2 -> Mux2/1
  Demux1/3 -> Mux2/2
  Mux2/1 -> To Workspace1/1
  "wdotTF "/1 -> Demux1/1
  w_meas/1 -> "wdotTF "/1
  Constant2/1 -> Mux/2
  Constant1/1 -> Mux/3
  Constant3/1 -> Mux/4

== matlab function Journal2022/SIKLEARN NETWORK/predictor 50 window ==
  data: BestSlip_SKlearn output; slip_buffer input; mu_buffer input
function BestSlip_SKlearn= fcn(slip_buffer, mu_buffer)
%#codegen

coder.extrinsic('py.wrapper_e86eb65e_MLPR_c50e1006.predict')
coder.extrinsic('py.numpy.array')
slip = slip_buffer;
mu = mu_buffer;
row_dataset = reshape([slip mu]',[],1);
npA = py.numpy.array(row_dataset(:).');

BestSlip_SKlearn = 0.0;

BestSlip_SKlearn = py.wrapper_e86eb65e_MLPR_c50e1006.predict([npA]);

== matlab function Journal2022/Aricraft Model/MATLAB Function ==
  data: mmu input; x input; xp output; M input; J input; Fz input; r input; Tw input
function xp = fcn(mmu,x,M,J,Fz,r,Tw)

v=x(1);
omega=x(2);

vp=-mmu*Fz/M;

omegap=(r*mmu*Fz-Tw)/J;

lambda=(v-omega*r)/v;

xp=[vp,omegap];

== matlab function Journal2022/Stima mu deriv2/mu estimation block ==
  data: vdot input; wdot input; torque_req input; mu_est output; phy_param input
function mu_est  = fcn(vdot, wdot, torque_req, phy_param)

%Nominal values loaded from file "Variables_Values -> phy_param muxed port"

M_vehicle = phy_param(1) ;      % Mass of aircraft(Kg) 
r =  phy_param(2)        ;      % radius of wheel (m)
J = phy_param(3)         ;      % Moment of Inertia of wheels (Kg * m^2) 
Fz = phy_param(4)        ;      % Normal force on  wheels (Newton)

%Meand of Fx from model
Fx1 = abs((J*wdot + torque_req)/r ); %%creava cambio di segno!
Fx2 = -(M_vehicle*vdot);
mu_est = ((Fx1+Fx2)/2)/Fz;
% mu_est = Fx2/Fz;

end

== matlab function Journal2022/Slip calc ==
  data: r input; v input; lambda output; w input
function lambda = fcn(r, v, w)
% longitudinal slip calc
lambda = (v-w*r)/v ;

== matlab function Journal2022/MATLAB Function1 ==
  data: vmin_stop input; v input; y output
function y = fcn(vmin_stop, v)
%
if v < vmin_stop
    
   y = 1;
   
else
    y= 0;

end
end

== matlab function Journal2022/PYTORCH NETWORKS/ DROPOUT ==
  data: bestSlip_NODO output; slip_buffer input; mu_buffer input; bestSlip_DO output; devStd_DO output
function [bestSlip_NODO ,bestSlip_DO, devStd_DO] = fcn(slip_buffer, mu_buffer)
%#codegen

coder.extrinsic('py.wrapper_Pytorch.predict')
coder.extrinsic('py.numpy.array')
slip = slip_buffer;
mu = mu_buffer;
row_dataset = reshape([slip mu]',[],1);
npA = py.numpy.array(row_dataset(:).');
bestSlip_NODO = 0.0;
bestSlip_DO = 0.0;
devStd_DO = 0.0;
out = double(py.wrapper_Pytorch.predict([npA]));
bestSlip_NODO = out(1);
bestSlip_DO = out(2);
devStd_DO = out(3);

== matlab function Journal2022/Aricraft Model/Burchkardt Road Model ==
  data: mu_slip output; lambda input; b1 input; best_slip output; mu_max output; b2 input; b3 input; lambda_dummy input
function [ mu_slip, best_slip,mu_max]= fcn(lambda,b1, b2, b3, lambda_dummy )
%#codegen
  

    mu_funct = [b1*(1-exp(-lambda_dummy*b2))-lambda_dummy*b3];
    [~, idx]= max(mu_funct);

    best_slip = lambda_dummy(idx);
    mu_max =  max(mu_funct);
    
    mu_slip =  b1*(1-exp(-lambda*b2))-lambda*b3;
    
   
  
end

== matlab function Journal2022/Aricraft Model/Pacejka Road  Model ==
  data: lambda_dummy input; lambda input; B input; C input; D input; E input; mu_slip output; best_slip output; mu_max output
function [mu_slip, best_slip,mu_max]= fcn(lambda_dummy,lambda,B,C,D,E)
% the tyre Model Provide a steady-state characteristic function, Fx=f(lambda,Fz)
% the longitudinal force Fx on the tire, based on:
% - Vertical load: Fz
% - Wheel slip: lambda
    
    fx_funct = D*sin(C*atan(B*lambda_dummy-E*(B*lambda_dummy-atan(B*lambda_dummy))));
    [~, idx]= max(fx_funct);
    best_slip = lambda_dummy(idx);
    mu_max =  max(fx_funct);
    
    mu_slip = D*sin(C*atan(B*lambda-E*(B*lambda-atan(B*lambda))));

== matlab function Journal2022/Aricraft Model/MATLAB Function2 ==
  data: omega input; v input; lambda output; r input
function lambda = fcn(omega,v, r)

lambda=(v-omega*r)/v;

== matlab function Journal2022/RLS ESTIMATE/RLS Best slip calc ==
  data: Thetas input; lambda_dummy input; bestslip output
function bestslip = fcn(Thetas, lambda_dummy)


mu_funct = Thetas(1)+ Thetas(2)*lambda_dummy + Thetas(3)*exp(-4.99*lambda_dummy)+ ...
    Thetas(4)*exp(-18.43*lambda_dummy) + Thetas(5)*exp(-65.62*lambda_dummy);
    [~, idx]= max(mu_funct);
    
bestslip = lambda_dummy(idx);
